simulink model "DFADAS2_SenFus_v1_201204RC_training_210115"  (R2018b)
settings: Solver=FixedStepDiscrete  StartTime=0.0  StopTime=inf  FixedStep=0.002  RelTol=1e-3  EnableMultiTasking=on
PreLoadFcn:
  | RTWConfigurationCB('preloadfcn', bdroot);
libraries: canmsglib x108, simulink x48, canfdmsglib x12
(part 9 of 28)

== system DFADAS2_SenFus_v1_201204RC_training_210115/Signal Input (Input)/Signal Input (50ms) (Input50)/Cmr/CmrInfo ==
  note: Level: 3
  Bus Creator : BusCreator  Inputs=6
  Bus Creator1 : BusCreator  Inputs=6
  Bus Creator2 : BusCreator  Inputs=5
  Bus Creator3 : BusCreator  Inputs=5
  Bus Creator4 : BusCreator  Inputs=4
  Bus Creator5 : BusCreator  Inputs=4
  "L0 Information (L0Info) " : Subsystem
  L1 Information (L1Info) : Subsystem
  R0 Information (R0Info) : Subsystem
  R1 Information (R1Info) : Subsystem
  LaneRx_bsLaneInfo : Outport
  LaneRx_efLanesFaultSyn : Outport  Port=2
  wires:
  Bus Creator/1 -> Bus Creator4/1  "CmrRxPrcs_bsL0Info"
  Bus Creator5/1 -> LaneRx_efLanesFaultSyn/1
  L1 Information (L1Info)/6(L1Info_efL1FaultSyn) -> Bus Creator5/3  "CmrRxPrcs_efL1FaultSyn"
  R0 Information (R0Info)/6(R0Info_facmR0Rng) -> Bus Creator1/6  "CmrRxPrcs_facmR0Rng"
  R1 Information (R1Info)/6(R0Info_efR0FaultSyn) -> Bus Creator5/4  "CmrRxPrcs_efR1FaultSyn"
  Bus Creator4/1 -> LaneRx_bsLaneInfo/1
  "L0 Information (L0Info) "/6(L0Info_facmL0Rng) -> Bus Creator/6  "CmrRxPrcs_facmL0Rng"
  R0 Information (R0Info)/4(R0Info_facmR0C3) -> Bus Creator1/4  "CmrRxPrcs_facmR0C3"
  R1 Information (R1Info)/1(R0Info_facmR0C0) -> Bus Creator3/1  "CmrRxPrcs_facmR1C0"
  R0 Information (R0Info)/3(R0Info_facmR0C2) -> Bus Creator1/3  "CmrRxPrcs_facmR0C2"
  "L0 Information (L0Info) "/4(L0Info_facmL0C3) -> Bus Creator/4  "CmrRxPrcs_facmL0C3"
  Bus Creator3/1 -> Bus Creator4/4  "CmrRxPrcs_bsR1Info"
  R0 Information (R0Info)/1(R0Info_facmR0C0) -> Bus Creator1/1  "CmrRxPrcs_facmR0C0"
  L1 Information (L1Info)/5(L1Info_facmL1Ql) -> Bus Creator2/5  "CmrRxPrcs_facmL1Ql"
  L1 Information (L1Info)/4(L1Info_facmL1C3) -> Bus Creator2/4  "CmrRxPrcs_facmL1C3"
  L1 Information (L1Info)/3(L1Info_facmL1C2) -> Bus Creator2/3  "CmrRxPrcs_facmL1C2"
  R0 Information (R0Info)/7(R0Info_efR0FaultSyn) -> Bus Creator5/2  "CmrRxPrcs_efR0FaultSyn"
  L1 Information (L1Info)/2(L1Info_facmL1C1) -> Bus Creator2/2  "CmrRxPrcs_facmL1C1"
  "L0 Information (L0Info) "/7(L0Info_efL0FaultSyn) -> Bus Creator5/1  "CmrRxPrcs_efL0FaultSyn"
  "L0 Information (L0Info) "/3(L0Info_facmL0C2) -> Bus Creator/3  "CmrRxPrcs_facmL0C2"
  R1 Information (R1Info)/4(R0Info_facmR0C3) -> Bus Creator3/4  "CmrRxPrcs_facmR1C3"
  R1 Information (R1Info)/2(R0Info_facmR0C1) -> Bus Creator3/2  "CmrRxPrcs_facmR1C1"
  Bus Creator2/1 -> Bus Creator4/3  "CmrRxPrcs_bsL1Info"
  R1 Information (R1Info)/3(R0Info_facmR0C2) -> Bus Creator3/3  "CmrRxPrcs_facmR1C2"
  "L0 Information (L0Info) "/1(L0Info_facmL0C0) -> Bus Creator/1  "CmrRxPrcs_facmL0C0"
  R0 Information (R0Info)/5(R0Info_facmR0Ql) -> Bus Creator1/5  "CmrRxPrcs_facmR0Ql"
  L1 Information (L1Info)/1(L1Info_facmL1C0) -> Bus Creator2/1  "CmrRxPrcs_facmL1C0"
  "L0 Information (L0Info) "/5(L0Info_facmL0Ql) -> Bus Creator/5  "CmrRxPrcs_facmL0Ql"
  "L0 Information (L0Info) "/2(L0Info_facmL0C1) -> Bus Creator/2  "CmrRxPrcs_facmL0C1"
  R1 Information (R1Info)/5(R0Info_facmR0Ql) -> Bus Creator3/5  "CmrRxPrcs_facmR1Ql"
  Bus Creator1/1 -> Bus Creator4/2  "CmrRxPrcs_bsR0Info"
  R0 Information (R0Info)/2(R0Info_facmR0C1) -> Bus Creator1/2  "CmrRxPrcs_facmR0C1"

== system DFADAS2_SenFus_v1_201204RC_training_210115/Signal Input (Input)/Signal Input (50ms) (Input50)/Front Left Radar(S2) Objects Information (FLRdr)/S0 Data Frame Read ==
  note: 目标：
      | ① 将可见的数据帧全部读出；
      | ② 仅对最新可见VF的数据帧进行数据解析。
      |
      | 首先将旧VF帧读完（不解析），然后进行RemainderCnt+1次的读取。最后一次读取的数据不解析，用于为未收到信号的通道置零。
  HFVFCnt : Inport
  IC : Inport  Port=2
  ObjectNum : Inport  Port=3
  Compare To Constant : simulink/Logic and Bit Operations/Compare To Constant  relop=>  const=0  OutDataTypeStr=boolean
  Enabled Subsystem : Subsystem  TreatAsAtomicUnit=on
  Logical Operator1 : Logic  Operator=OR  AllPortsSameDT=off  OutDataTypeStr=boolean
  Logical Operator3 : Logic  AllPortsSameDT=off  OutDataTypeStr=boolean
  Relational Operator3 : RelationalOperator  Operator===  OutDataTypeStr=boolean  RndMeth=Simplest
  S-Function200 : S-Function  FunctionName=NSTC297CANFDReceiveBlkLib  Parameters=|  SFunctionDeploymentMode=off  EnableBusSupport=off  mask(NSTC297 CANFD Receive){Ns_DeviceID=General Control Unit Gen2, Ns_ChannelNum=1, Ns_FrameID=855, Ns_IsVirtualFrame=on, Ns_RoleInVirtualFrame=Data Frame, Ns_HeaderFrameID=854, Ns_VirtualFrameStatusFlg=off, Ns_IncompleteFrameCntFlg=off, Ns_OverflowCntFlg=off, Ns_FrameBufferSize=5, Ns_SampleTime=-1}
      | uint16(Ns_DeviceID),
      | uint16(Ns_ChannelNum),
      | uint32(Ns_FrameID),
      | uint8(Ns_IsVirtualFrame),
      | uint16(Ns_RoleInVirtualFrame),
      | uint32(Ns_HeaderFrameID),
      | uint8(Ns_VirtualFrameStatusFlg),
      | uint8(Ns_IncompleteFrameCntFlg),
      | uint8(Ns_OverflowCntFlg),
      | uint16(Ns_FrameBufferSize),
      | double(Ns_SampleTime)
      mask prompts: Ns_DeviceID "Device:"; Ns_ChannelNum "Channel number:"; Ns_FrameID "Frame ID:"; Ns_IsVirtualFrame "Belong to a virtual frame"; Ns_RoleInVirtualFrame "Position in virtual frame:"; Ns_HeaderFrameID "Header frame ID:"; Ns_VirtualFrameStatusFlg "Current virtural frame status output"; Ns_IncompleteFrameCntFlg "Incomplete virtual frame count output"; Ns_OverflowCntFlg "Overflow count output"; Ns_FrameBufferSize "Frame buffer size:"; Ns_SampleTime "Sample time:"
      mask init:
      | NSTC297CANFDReceive_callback('portlabels');
      mask TypeOptions Ns_DeviceID: General Control Unit Gen2 | ADAS Control Unit Gen2
      mask TypeOptions Ns_ChannelNum: 0 | 1 | 2 | 3 | 4 | 5
      mask Callback Ns_IsVirtualFrame: NSTC297CANFDReceive_callback('Belong to a virtual frame');
      mask TypeOptions Ns_RoleInVirtualFrame: Header Frame | Data Frame | Trailer Frame
      mask Callback Ns_RoleInVirtualFrame: NSTC297CANFDReceive_callback('Position in virtual frame');
      mask Display: color('blue');text(0.02,0.9,'NovSteeds TC297','horizontalAlignment','left');color('blue');text(0.5,0.7,'CANFD Receive','horizontalAlignment','center');color('black');text(0.5,0.6,'Channel: 1','horizontalAlignment','center');text(0.5,0.5,'ID: 855','horizontalAlignment','center');text(0.5,0.4,'Virtual Frame: Data Frame','horizontalAlignment','center');port_label('output',1, 'VFCnt');port_label('output',2, 'RemainderCnt');port_label('output',3, 'Msg');
  Subsystem : Subsystem
  Switch : Switch  Criteria=u2 > Threshold
  VsblMnmt : Subsystem
  While Iterator : WhileIterator  MaxIters=10  ResetStates=reset
  RLRdr_bsObjInfo : Outport
  wires:
  Switch/1 -> RLRdr_bsObjInfo/1
  ObjectNum/1 -> Switch/2, Enabled Subsystem/3(obj_num)
  Logical Operator3/1 -> Enabled Subsystem/Enable, Logical Operator1/2
  Subsystem/1(RLRdrObjInfo) -> Switch/3
  Enabled Subsystem/1(RLRdrObjInfo) -> Switch/1
  Compare To Constant/1 -> Logical Operator3/2
  Relational Operator3/1 -> Logical Operator3/1
  Logical Operator1/1 -> While Iterator/1
  VsblMnmt/1(EnFlg) -> Logical Operator1/1
  HFVFCnt/1 -> Relational Operator3/1, VsblMnmt/1(HFVFCnt)
  S-Function200/1 -> Relational Operator3/2, VsblMnmt/2(LocVFCnt)
  S-Function200/2 -> Enabled Subsystem/1(RemainderCnt), Compare To Constant/1
  S-Function200/3 -> Enabled Subsystem/2(Msg)
  IC/1 -> While Iterator/2

== system DFADAS2_SenFus_v1_201204RC_training_210115/Signal Input (Input)/Signal Input (50ms) (Input50)/Front Left Radar(S2) Objects Information (FLRdr)/S0 Header Frame Read ==
  note: 目标：
      | ① 将缓冲中的全部数据读出；
      | ② 仅对最后一帧进行解析
  IC : Inport
  Compare To Constant : simulink/Logic and Bit Operations/Compare To Constant  relop=>  const=0  OutDataTypeStr=boolean
  Compare To Constant1 : simulink/Logic and Bit Operations/Compare To Constant  relop===  const=1  OutDataTypeStr=boolean
  Enabled Subsystem : Subsystem  TreatAsAtomicUnit=on
  S-Function100 : S-Function  FunctionName=NSTC297CANFDReceiveBlkLib  Parameters=|  SFunctionDeploymentMode=off  EnableBusSupport=off  mask(NSTC297 CANFD Receive){Ns_DeviceID=General Control Unit Gen2, Ns_ChannelNum=1, Ns_FrameID=854, Ns_IsVirtualFrame=on, Ns_RoleInVirtualFrame=Header Frame, Ns_HeaderFrameID=0, Ns_VirtualFrameStatusFlg=off, Ns_IncompleteFrameCntFlg=off, Ns_OverflowCntFlg=off, Ns_FrameBufferSize=5, Ns_SampleTime=-1}
      | uint16(Ns_DeviceID),
      | uint16(Ns_ChannelNum),
      | uint32(Ns_FrameID),
      | uint8(Ns_IsVirtualFrame),
      | uint16(Ns_RoleInVirtualFrame),
      | uint32(Ns_HeaderFrameID),
      | uint8(Ns_VirtualFrameStatusFlg),
      | uint8(Ns_IncompleteFrameCntFlg),
      | uint8(Ns_OverflowCntFlg),
      | uint16(Ns_FrameBufferSize),
      | double(Ns_SampleTime)
      mask prompts: Ns_DeviceID "Device:"; Ns_ChannelNum "Channel number:"; Ns_FrameID "Frame ID:"; Ns_IsVirtualFrame "Belong to a virtual frame"; Ns_RoleInVirtualFrame "Position in virtual frame:"; Ns_HeaderFrameID "Header frame ID:"; Ns_VirtualFrameStatusFlg "Current virtural frame status output"; Ns_IncompleteFrameCntFlg "Incomplete virtual frame count output"; Ns_OverflowCntFlg "Overflow count output"; Ns_FrameBufferSize "Frame buffer size:"; Ns_SampleTime "Sample time:"
      mask init:
      | NSTC297CANFDReceive_callback('portlabels');
      mask TypeOptions Ns_DeviceID: General Control Unit Gen2 | ADAS Control Unit Gen2
      mask TypeOptions Ns_ChannelNum: 0 | 1 | 2 | 3 | 4 | 5
      mask Callback Ns_IsVirtualFrame: NSTC297CANFDReceive_callback('Belong to a virtual frame');
      mask TypeOptions Ns_RoleInVirtualFrame: Header Frame | Data Frame | Trailer Frame
      mask Callback Ns_RoleInVirtualFrame: NSTC297CANFDReceive_callback('Position in virtual frame');
      mask Display: color('blue');text(0.02,0.9,'NovSteeds TC297','horizontalAlignment','left');color('blue');text(0.5,0.7,'CANFD Receive','horizontalAlignment','center');color('black');text(0.5,0.6,'Channel: 1','horizontalAlignment','center');text(0.5,0.5,'ID: 854','horizontalAlignment','center');text(0.5,0.4,'Virtual Frame: Header Frame','horizontalAlignment','center');port_label('output',1, 'VFCnt');port_label('output',2, 'RemainderCnt');port_label('output',3, 'Msg');
  While Iterator : WhileIterator  MaxIters=10  ResetStates=reset
  RLRdr_bsCmnInfo : Outport
  HFVFCnt : Outport  Port=2
  wires:
  S-Function100/1 -> HFVFCnt/1
  Compare To Constant1/1 -> Enabled Subsystem/Enable
  S-Function100/2 -> Compare To Constant1/1, Compare To Constant/1
  Enabled Subsystem/1(Sigs) -> RLRdr_bsCmnInfo/1
  S-Function100/3 -> Enabled Subsystem/1(Msg)
  Compare To Constant/1 -> While Iterator/1
  IC/1 -> While Iterator/2

== system DFADAS2_SenFus_v1_201204RC_training_210115/Signal Input (Input)/Signal Input (50ms) (Input50)/Front Left Radar(S2) Objects Information (FLRdr)/S0 Trailer Frame Read ==
  HFVFCnt : Inport
  "IC " : Inport  Port=2
  S-Function300 : S-Function  FunctionName=NSTC297CANFDReceiveBlkLib  Parameters=|  SFunctionDeploymentMode=off  EnableBusSupport=off  mask(NSTC297 CANFD Receive){Ns_DeviceID=General Control Unit Gen2, Ns_ChannelNum=1, Ns_FrameID=856, Ns_IsVirtualFrame=on, Ns_RoleInVirtualFrame=Trailer Frame, Ns_HeaderFrameID=854, Ns_VirtualFrameStatusFlg=off, Ns_IncompleteFrameCntFlg=off, Ns_OverflowCntFlg=off, Ns_FrameBufferSize=5, Ns_SampleTime=-1}
      | uint16(Ns_DeviceID),
      | uint16(Ns_ChannelNum),
      | uint32(Ns_FrameID),
      | uint8(Ns_IsVirtualFrame),
      | uint16(Ns_RoleInVirtualFrame),
      | uint32(Ns_HeaderFrameID),
      | uint8(Ns_VirtualFrameStatusFlg),
      | uint8(Ns_IncompleteFrameCntFlg),
      | uint8(Ns_OverflowCntFlg),
      | uint16(Ns_FrameBufferSize),
      | double(Ns_SampleTime)
      mask prompts: Ns_DeviceID "Device:"; Ns_ChannelNum "Channel number:"; Ns_FrameID "Frame ID:"; Ns_IsVirtualFrame "Belong to a virtual frame"; Ns_RoleInVirtualFrame "Position in virtual frame:"; Ns_HeaderFrameID "Header frame ID:"; Ns_VirtualFrameStatusFlg "Current virtural frame status output"; Ns_IncompleteFrameCntFlg "Incomplete virtual frame count output"; Ns_OverflowCntFlg "Overflow count output"; Ns_FrameBufferSize "Frame buffer size:"; Ns_SampleTime "Sample time:"
      mask init:
      | NSTC297CANFDReceive_callback('portlabels');
      mask TypeOptions Ns_DeviceID: General Control Unit Gen2 | ADAS Control Unit Gen2
      mask TypeOptions Ns_ChannelNum: 0 | 1 | 2 | 3 | 4 | 5
      mask Callback Ns_IsVirtualFrame: NSTC297CANFDReceive_callback('Belong to a virtual frame');
      mask TypeOptions Ns_RoleInVirtualFrame: Header Frame | Data Frame | Trailer Frame
      mask Callback Ns_RoleInVirtualFrame: NSTC297CANFDReceive_callback('Position in virtual frame');
      mask Display: color('blue');text(0.02,0.9,'NovSteeds TC297','horizontalAlignment','left');color('blue');text(0.5,0.7,'CANFD Receive','horizontalAlignment','center');color('black');text(0.5,0.6,'Channel: 1','horizontalAlignment','center');text(0.5,0.5,'ID: 856','horizontalAlignment','center');text(0.5,0.4,'Virtual Frame: Trailer Frame','horizontalAlignment','center');port_label('output',1, 'VFCnt');port_label('output',2, 'RemainderCnt');port_label('output',3, 'Msg');
  Terminator1 : Terminator
  Terminator2 : Terminator
  VsblMnmt : Subsystem
  While Iterator : WhileIterator  MaxIters=10  ResetStates=reset
  wires:
  VsblMnmt/1(EnFlg) -> While Iterator/1
  S-Function300/1 -> VsblMnmt/2(LocVFCnt)
  HFVFCnt/1 -> VsblMnmt/1(HFVFCnt)
  S-Function300/2 -> Terminator2/1
  S-Function300/3 -> Terminator1/1
  "IC "/1 -> While Iterator/2

== system DFADAS2_SenFus_v1_201204RC_training_210115/Signal Input (Input)/Signal Input (50ms) (Input50)/Front Left Radar(S2) Objects Information (FLRdr)/Subsystem ==
  In1 : Inport
  Bus Selector : BusSelector  OutputSignals=FLRdr_bsObjInfo.M00ObjInfo,FLRdr_bsObjInfo.M01ObjInfo,FLRdr_bsObjInfo.M10ObjInfo,FLRdr_bsObjInfo.M11ObjInfo,FLRdr_bsObjInfo.M20ObjInfo,FLRdr_bsObjInfo.M21ObjInfo,FLRdr_bsObjInfo.M30ObjInfo,FLRdr_bsObjInfo.M31ObjInfo,FLRdr_bsObjInfo.M40ObjInfo,FLRdr_bsObjInfo.M41ObjInfo,FLRdr_bsCmnInfo
  Bus Selector1 : BusSelector  OutputSignals=Id_S0_001,XPos_S0_001,YPos_S0_001
  Bus Selector10 : BusSelector  OutputSignals=Id_S0_008,XPos_S0_008,YPos_S0_008
  Bus Selector11 : BusSelector  OutputSignals=Id_S0_009,XPos_S0_009,YPos_S0_009
  Bus Selector2 : BusSelector  OutputSignals=Id_S0_002,XPos_S0_002,YPos_S0_002
  Bus Selector3 : BusSelector  OutputSignals=Id_S0_003,XPos_S0_003,YPos_S0_003
  Bus Selector4 : BusSelector  OutputSignals=Id_S0_004,XPos_S0_004,YPos_S0_004
  Bus Selector5 : BusSelector  OutputSignals=Id_S0_005,XPos_S0_005,YPos_S0_005
  Bus Selector6 : BusSelector  OutputSignals=NumberOfObjects_S2
  Bus Selector7 : BusSelector  OutputSignals=Id_S0_010,XPos_S0_010,YPos_S0_010
  Bus Selector8 : BusSelector  OutputSignals=Id_S0_006,XPos_S0_006,YPos_S0_006
  Bus Selector9 : BusSelector  OutputSignals=Id_S0_007,XPos_S0_007,YPos_S0_007
  CAN FD Pack : canfdmsglib/CAN FD Pack  MsgList=(none)  MsgName=Msg  ProtocolMode=CAN FD  MsgIDType=Standard (11-bit identifier)  MsgIdentifier=1634  MsgLength=64  SignalInfo=Signal1$0$16$1$2$1$0$1$0$0$Inf$#Signal2$16$16$1$2$1$0$0.05$-400$-Inf$Inf$#Signal3$32$16$1$2$1$0$0.01$-80$-Inf$Inf$#Signal4$48$16$1$2$1$0$1$0$0$Inf$#Signal5$64$16$1$2$1$0$0.05$-400$-Inf$Inf$#Signal6$80$16$1$2$1$0$0.01$-80$-Inf$Inf$#Signal7$96$16$1$2$1$0$1$0$0$Inf$#Signal8$112$16$1$2$1$0$0.05$-400$-Inf$Inf$#Signal9$128$16$1$2$1$0$0.01$-80$-Inf$Inf$#Signal10$144$16$1$2$1$0$1$0$0$Inf$#Signal11$160$16$1$2$1$0$0.05$-400$-Inf$Inf$#Signal12$176$16$1$2$1$0$0.01$-80$-Inf$Inf$#Signal13$192$16$1$2$1$0$1$0$0$Inf$#Signal14$208$16$1$2$1$0$0.05$-400$-Inf$Inf$#Signal15$224$16$1$2$1$0$0.01$-80$-Inf$Inf$#Signal16$240$16$1$2$1$0$1$0$0$Inf$#Signal17$256$16$1$2$1$0$0.05$-400$-Inf$Inf$#Signal18$272$16$1$2$1$0$0.01$-80$-Inf$Inf$#Signal19$288$16$1$2$1$0$1$0$0$Inf$#Signal20$304$16$1$2$1$0$0.05$-400$-Inf$Inf$#Signal21$320$16$1$2$1$0$0.01$-80$-Inf$Inf$#Signal22$336$16$1$2$1$0$1$0$0$Inf$#Signal23$352$16$1$2$1$0$0.05$-400$-Inf$Inf$#Signal24$368$16$1$2$1$0$0.01$-80$-Inf$Inf$#Signal25$384$16$1$2$1$0$1$0$0$Inf$#Signal26$400$16$1$2$1$0$0.05$-400$-Inf$Inf$#Signal27$416$16$1$2$1$0$0.01$-80$-Inf$Inf$#Signal28$432$16$1$2$1$0$1$0$0$Inf$#Signal29$448$16$1$2$1$0$0.05$-400$-Inf$Inf$#Signal30$464$16$1$2$1$0$0.01$-80$-Inf$Inf$#num_obj$480$16$1$2$1$0$1$0$0$Inf$#m_value$496$16$1$2$1$0$1$0$0$Inf$#  NSignals=32  StartBits=str2num('[int32(0);int32(16);int32(32);int32(48);int32(64);int32(80);int32(96);int32(112);int32(128);int32(144);int32(160);int32(176);int32(192);int32(208);int32(224);int32(240);int32(256);int32(272);int32(288);int32(304);int32(320);int32(336);int32(352);int32(368);int32(384);int32(400);int32(416);int32(432);int32(448);int32(464);int32(480);int32(496)]')  SignalSizes=str2num('[int32(16);int32(16);int32(16);int32(16);int32(16);int32(16);int32(16);int32(16);int32(16);int32(16);int32(16);int32(16);int32(16);int32(16);int32(16);int32(16);int32(16);int32(16);int32(16);int32(16);int32(16);int32(16);int32(16);int32(16);int32(16);int32(16);int32(16);int32(16);int32(16);int32(16);int32(16);int32(16)]')  ByteOrders=str2num('[int32(1);int32(1);int32(1);int32(1);int32(1);int32(1);int32(1);int32(1);int32(1);int32(1);int32(1);int32(1);int32(1);int32(1);int32(1);int32(1);int32(1);int32(1);int32(1);int32(1);int32(1);int32(1);int32(1);int32(1);int32(1);int32(1);int32(1);int32(1);int32(1);int32(1);int32(1);int32(1)]')  DataTypes=str2num('[int32(2);int32(2);int32(2);int32(2);int32(2);int32(2);int32(2);int32(2);int32(2);int32(2);int32(2);int32(2);int32(2);int32(2);int32(2);int32(2);int32(2);int32(2);int32(2);int32(2);int32(2);int32(2);int32(2);int32(2);int32(2);int32(2);int32(2);int32(2);int32(2);int32(2);int32(2);int32(2)]')  MultiplexTypes=str2num('[int32(1);int32(1);int32(1);int32(1);int32(1);int32(1);int32(1);int32(1);int32(1);int32(1);int32(1);int32(1);int32(1);int32(1);int32(1);int32(1);int32(1);int32(1);int32(1);int32(1);int32(1);int32(1);int32(1);int32(1);int32(1);int32(1);int32(1);int32(1);int32(1);int32(1);int32(1);int32(1)]')  MultiplexValues=str2num('[double(0);double(0);double(0);double(0);double(0);double(0);double(0);double(0);double(0);double(0);double(0);double(0);double(0);double(0);double(0);double(0);double(0);double(0);double(0);double(0);double(0);double(0);double(0);double(0);double(0);double(0);double(0);double(0);double(0);double(0);double(0);double(0)]')  Factors=str2num('[double(1);double(0.05);double(0.01);double(1);double(0.05);double(0.01);double(1);double(0.05);double(0.01);double(1);double(0.05);double(0.01);double(1);double(0.05);double(0.01);double(1);double(0.05);double(0.01);double(1);double(0.05);double(0.01);double(1);double(0.05);double(0.01);double(1);double(0.05);double(0.01);double(1);double(0.05);double(0.01);double(1);double(1)]')  Offsets=str2num('[double(0);double(-400);double(-80);double(0);double(-400);double(-80);double(0);double(-400);double(-80);double(0);double(-400);double(-80);double(0);double(-400);double(-80);double(0);double(-400);double(-80);double(0);double(-400);double(-80);double(0);double(-400);double(-80);double(0);double(-400);double(-80);double(0);double(-400);double(-80);double(0);double(0)]')  Minimums=str2num('[double(0);double(-Inf);double(-Inf);double(0);double(-Inf);double(-Inf);double(0);double(-Inf);double(-Inf);double(0);double(-Inf);double(-Inf);double(0);double(-Inf);double(-Inf);double(0);double(-Inf);double(-Inf);double(0);double(-Inf);double(-Inf);double(0);double(-Inf);double(-Inf);double(0);double(-Inf);double(-Inf);double(0);double(-Inf);double(-Inf);double(0);double(0)]')  Maximums=str2num('[double(Inf);double(Inf);double(Inf);double(Inf);double(Inf);double(Inf);double(Inf);double(Inf);double(Inf);double(Inf);double(Inf);double(Inf);double(Inf);double(Inf);double(Inf);double(Inf);double(Inf);double(Inf);double(Inf);double(Inf);double(Inf);double(Inf);double(Inf);double(Inf);double(Inf);double(Inf);double(Inf);double(Inf);double(Inf);double(Inf);double(Inf);double(Inf)]')  Remote=off  ApplyMinMax=off  BRSSwitch=off
      settings: SourceProductName=Simulink Real-Time  DataFormat=manually specified signals
  S-Function9 : S-Function  FunctionName=NSTC297CANFDTransmitBlkLib  Parameters=|  SFunctionDeploymentMode=off  EnableBusSupport=off  mask(NSTC297 CANFD Transmit){Ns_DeviceID=ADAS Control Unit Gen2, Ns_ChannelNum=3, Ns_FrameType=CANFD, Ns_FrameBufferSize=0, Ns_OverflowCntOutFlg=off, Ns_SampleTime=-1}
      | uint16(Ns_DeviceID),
      | uint16(Ns_ChannelNum),
      | uint16(Ns_FrameType),
      | uint16(Ns_FrameBufferSize),
      | uint8(Ns_OverflowCntOutFlg),
      | double(Ns_SampleTime)
      mask prompts: Ns_DeviceID "Device:"; Ns_ChannelNum "Channel number:"; Ns_FrameType "Frame type:"; Ns_FrameBufferSize "Frame buffer size:"; Ns_OverflowCntOutFlg "Overflow count output"; Ns_SampleTime "Sample time:"
      mask init:
      | NSTC297CANFDTransmit_callback('portlabels');
      mask TypeOptions Ns_DeviceID: General Control Unit Gen2 | ADAS Control Unit Gen2
      mask TypeOptions Ns_ChannelNum: 0 | 1 | 2 | 3 | 4 | 5
      mask TypeOptions Ns_FrameType: CAN | CANFD
      mask Display: color('blue');text(0.98,0.9,'NovSteeds TC297','horizontalAlignment','right');color('blue');text(0.5,0.65,'CANFD Transmit','horizontalAlignment','center');color('black');text(0.5,0.35,'Type: CANFD','horizontalAlignment','center');text(0.5,0.50,'Channel: 3','horizontalAlignment','center');port_label('input',1, 'Msg');
  wires:
  Bus Selector/2 -> Bus Selector2/1  "<M01ObjInfo>"
  Bus Selector7/1 -> CAN FD Pack/28  "<Id_S0_010>"
  Bus Selector/11 -> Bus Selector6/1  "<FLRdr_bsCmnInfo>"
  Bus Selector6/1 -> CAN FD Pack/31  "<NumberOfObjects_S2>"
  Bus Selector8/3 -> CAN FD Pack/18  "<YPos_S0_006>"
  Bus Selector3/2 -> CAN FD Pack/8  "<XPos_S0_003>"
  Bus Selector7/3 -> CAN FD Pack/30  "<YPos_S0_010>"
  Bus Selector3/3 -> CAN FD Pack/9  "<YPos_S0_003>"
  Bus Selector9/3 -> CAN FD Pack/21  "<YPos_S0_007>"
  Bus Selector2/1 -> CAN FD Pack/4  "<Id_S0_002>"
  Bus Selector7/2 -> CAN FD Pack/29  "<XPos_S0_010>"
  Bus Selector10/1 -> CAN FD Pack/22  "<Id_S0_008>"
  In1/1 -> Bus Selector/1
  Bus Selector11/2 -> CAN FD Pack/26  "<XPos_S0_009>"
  Bus Selector10/2 -> CAN FD Pack/23  "<XPos_S0_008>"
  Bus Selector4/3 -> CAN FD Pack/12  "<YPos_S0_004>"
  Bus Selector2/3 -> CAN FD Pack/6  "<YPos_S0_002>"
  Bus Selector4/2 -> CAN FD Pack/11  "<XPos_S0_004>"
  Bus Selector1/1 -> CAN FD Pack/1  "<Id_S0_001>"
  CAN FD Pack/1 -> S-Function9/1
  Bus Selector8/1 -> CAN FD Pack/16  "<Id_S0_006>"
  Bus Selector5/2 -> CAN FD Pack/14  "<XPos_S0_005>"
  Bus Selector2/2 -> CAN FD Pack/5  "<XPos_S0_002>"
  Bus Selector11/3 -> CAN FD Pack/27  "<YPos_S0_009>"
  Bus Selector3/1 -> CAN FD Pack/7  "<Id_S0_003>"
  Bus Selector/6 -> Bus Selector8/1  "<M21ObjInfo>"
  Bus Selector5/3 -> CAN FD Pack/15  "<YPos_S0_005>"
  Bus Selector4/1 -> CAN FD Pack/10  "<Id_S0_004>"
  Bus Selector10/3 -> CAN FD Pack/24  "<YPos_S0_008>"
  Bus Selector/7 -> Bus Selector9/1  "<M30ObjInfo>"
  Bus Selector1/3 -> CAN FD Pack/3  "<YPos_S0_001>"
  Bus Selector/1 -> Bus Selector1/1  "<M00ObjInfo>"
  Bus Selector/9 -> Bus Selector11/1  "<M40ObjInfo>"
  Bus Selector/8 -> Bus Selector10/1  "<M31ObjInfo>"
  Bus Selector9/1 -> CAN FD Pack/19  "<Id_S0_007>"
  Bus Selector9/2 -> CAN FD Pack/20  "<XPos_S0_007>"
  Bus Selector/3 -> Bus Selector3/1  "<M10ObjInfo>"
  Bus Selector/5 -> Bus Selector5/1  "<M20ObjInfo>"
  Bus Selector/4 -> Bus Selector4/1  "<M11ObjInfo>"
  Bus Selector1/2 -> CAN FD Pack/2  "<XPos_S0_001>"
  Bus Selector5/1 -> CAN FD Pack/13  "<Id_S0_005>"
  Bus Selector11/1 -> CAN FD Pack/25  "<Id_S0_009>"
  Bus Selector8/2 -> CAN FD Pack/17  "<XPos_S0_006>"
  Bus Selector/10 -> Bus Selector7/1  "<M41ObjInfo>"

== system DFADAS2_SenFus_v1_201204RC_training_210115/Signal Input (Input)/Signal Input (50ms) (Input50)/Front Right Radar(S3) Objects Information (FRRdr)/S0 Data Frame Read ==
  note: 目标：
      | ① 将可见的数据帧全部读出；
      | ② 仅对最新可见VF的数据帧进行数据解析。
      |
      | 首先将旧VF帧读完（不解析），然后进行RemainderCnt+1次的读取。最后一次读取的数据不解析，用于为未收到信号的通道置零。
  HFVFCnt : Inport
  IC : Inport  Port=2
  ObjectNum : Inport  Port=3
  Compare To Constant : simulink/Logic and Bit Operations/Compare To Constant  relop=>  const=0  OutDataTypeStr=boolean
  Enabled Subsystem : Subsystem  TreatAsAtomicUnit=on
  Logical Operator1 : Logic  Operator=OR  AllPortsSameDT=off  OutDataTypeStr=boolean
  Logical Operator3 : Logic  AllPortsSameDT=off  OutDataTypeStr=boolean
  Relational Operator3 : RelationalOperator  Operator===  OutDataTypeStr=boolean  RndMeth=Simplest
  S-Function200 : S-Function  FunctionName=NSTC297CANFDReceiveBlkLib  Parameters=|  SFunctionDeploymentMode=off  EnableBusSupport=off  mask(NSTC297 CANFD Receive){Ns_DeviceID=General Control Unit Gen2, Ns_ChannelNum=1, Ns_FrameID=858, Ns_IsVirtualFrame=on, Ns_RoleInVirtualFrame=Data Frame, Ns_HeaderFrameID=857, Ns_VirtualFrameStatusFlg=off, Ns_IncompleteFrameCntFlg=off, Ns_OverflowCntFlg=off, Ns_FrameBufferSize=5, Ns_SampleTime=-1}
      | uint16(Ns_DeviceID),
      | uint16(Ns_ChannelNum),
      | uint32(Ns_FrameID),
      | uint8(Ns_IsVirtualFrame),
      | uint16(Ns_RoleInVirtualFrame),
      | uint32(Ns_HeaderFrameID),
      | uint8(Ns_VirtualFrameStatusFlg),
      | uint8(Ns_IncompleteFrameCntFlg),
      | uint8(Ns_OverflowCntFlg),
      | uint16(Ns_FrameBufferSize),
      | double(Ns_SampleTime)
      mask prompts: Ns_DeviceID "Device:"; Ns_ChannelNum "Channel number:"; Ns_FrameID "Frame ID:"; Ns_IsVirtualFrame "Belong to a virtual frame"; Ns_RoleInVirtualFrame "Position in virtual frame:"; Ns_HeaderFrameID "Header frame ID:"; Ns_VirtualFrameStatusFlg "Current virtural frame status output"; Ns_IncompleteFrameCntFlg "Incomplete virtual frame count output"; Ns_OverflowCntFlg "Overflow count output"; Ns_FrameBufferSize "Frame buffer size:"; Ns_SampleTime "Sample time:"
      mask init:
      | NSTC297CANFDReceive_callback('portlabels');
      mask TypeOptions Ns_DeviceID: General Control Unit Gen2 | ADAS Control Unit Gen2
      mask TypeOptions Ns_ChannelNum: 0 | 1 | 2 | 3 | 4 | 5
      mask Callback Ns_IsVirtualFrame: NSTC297CANFDReceive_callback('Belong to a virtual frame');
      mask TypeOptions Ns_RoleInVirtualFrame: Header Frame | Data Frame | Trailer Frame
      mask Callback Ns_RoleInVirtualFrame: NSTC297CANFDReceive_callback('Position in virtual frame');
      mask Display: color('blue');text(0.02,0.9,'NovSteeds TC297','horizontalAlignment','left');color('blue');text(0.5,0.7,'CANFD Receive','horizontalAlignment','center');color('black');text(0.5,0.6,'Channel: 1','horizontalAlignment','center');text(0.5,0.5,'ID: 858','horizontalAlignment','center');text(0.5,0.4,'Virtual Frame: Data Frame','horizontalAlignment','center');port_label('output',1, 'VFCnt');port_label('output',2, 'RemainderCnt');port_label('output',3, 'Msg');
  Subsystem : Subsystem
  Switch : Switch  Criteria=u2 > Threshold
  VsblMnmt : Subsystem
  While Iterator : WhileIterator  MaxIters=10  ResetStates=reset
  RLRdr_bsObjInfo : Outport
  wires:
  IC/1 -> While Iterator/2
  S-Function200/3 -> Enabled Subsystem/2(Msg)
  S-Function200/2 -> Compare To Constant/1, Enabled Subsystem/1(RemainderCnt)
  S-Function200/1 -> VsblMnmt/2(LocVFCnt), Relational Operator3/2
  HFVFCnt/1 -> VsblMnmt/1(HFVFCnt), Relational Operator3/1
  VsblMnmt/1(EnFlg) -> Logical Operator1/1
  Logical Operator1/1 -> While Iterator/1
  Relational Operator3/1 -> Logical Operator3/1
  Compare To Constant/1 -> Logical Operator3/2
  Enabled Subsystem/1(RLRdrObjInfo) -> Switch/1
  Subsystem/1(RLRdrObjInfo) -> Switch/3
  Logical Operator3/1 -> Logical Operator1/2, Enabled Subsystem/Enable
  ObjectNum/1 -> Enabled Subsystem/3(obj_num), Switch/2
  Switch/1 -> RLRdr_bsObjInfo/1

== system DFADAS2_SenFus_v1_201204RC_training_210115/Signal Input (Input)/Signal Input (50ms) (Input50)/Front Right Radar(S3) Objects Information (FRRdr)/S0 Header Frame Read ==
  note: 目标：
      | ① 将缓冲中的全部数据读出；
      | ② 仅对最后一帧进行解析
  IC : Inport
  Compare To Constant : simulink/Logic and Bit Operations/Compare To Constant  relop=>  const=0  OutDataTypeStr=boolean
  Compare To Constant1 : simulink/Logic and Bit Operations/Compare To Constant  relop===  const=1  OutDataTypeStr=boolean
  Enabled Subsystem : Subsystem  TreatAsAtomicUnit=on
  S-Function100 : S-Function  FunctionName=NSTC297CANFDReceiveBlkLib  Parameters=|  SFunctionDeploymentMode=off  EnableBusSupport=off  mask(NSTC297 CANFD Receive){Ns_DeviceID=General Control Unit Gen2, Ns_ChannelNum=1, Ns_FrameID=857, Ns_IsVirtualFrame=on, Ns_RoleInVirtualFrame=Header Frame, Ns_HeaderFrameID=0, Ns_VirtualFrameStatusFlg=off, Ns_IncompleteFrameCntFlg=off, Ns_OverflowCntFlg=off, Ns_FrameBufferSize=5, Ns_SampleTime=-1}
      | uint16(Ns_DeviceID),
      | uint16(Ns_ChannelNum),
      | uint32(Ns_FrameID),
      | uint8(Ns_IsVirtualFrame),
      | uint16(Ns_RoleInVirtualFrame),
      | uint32(Ns_HeaderFrameID),
      | uint8(Ns_VirtualFrameStatusFlg),
      | uint8(Ns_IncompleteFrameCntFlg),
      | uint8(Ns_OverflowCntFlg),
      | uint16(Ns_FrameBufferSize),
      | double(Ns_SampleTime)
      mask prompts: Ns_DeviceID "Device:"; Ns_ChannelNum "Channel number:"; Ns_FrameID "Frame ID:"; Ns_IsVirtualFrame "Belong to a virtual frame"; Ns_RoleInVirtualFrame "Position in virtual frame:"; Ns_HeaderFrameID "Header frame ID:"; Ns_VirtualFrameStatusFlg "Current virtural frame status output"; Ns_IncompleteFrameCntFlg "Incomplete virtual frame count output"; Ns_OverflowCntFlg "Overflow count output"; Ns_FrameBufferSize "Frame buffer size:"; Ns_SampleTime "Sample time:"
      mask init:
      | NSTC297CANFDReceive_callback('portlabels');
      mask TypeOptions Ns_DeviceID: General Control Unit Gen2 | ADAS Control Unit Gen2
      mask TypeOptions Ns_ChannelNum: 0 | 1 | 2 | 3 | 4 | 5
      mask Callback Ns_IsVirtualFrame: NSTC297CANFDReceive_callback('Belong to a virtual frame');
      mask TypeOptions Ns_RoleInVirtualFrame: Header Frame | Data Frame | Trailer Frame
      mask Callback Ns_RoleInVirtualFrame: NSTC297CANFDReceive_callback('Position in virtual frame');
      mask Display: color('blue');text(0.02,0.9,'NovSteeds TC297','horizontalAlignment','left');color('blue');text(0.5,0.7,'CANFD Receive','horizontalAlignment','center');color('black');text(0.5,0.6,'Channel: 1','horizontalAlignment','center');text(0.5,0.5,'ID: 857','horizontalAlignment','center');text(0.5,0.4,'Virtual Frame: Header Frame','horizontalAlignment','center');port_label('output',1, 'VFCnt');port_label('output',2, 'RemainderCnt');port_label('output',3, 'Msg');
  While Iterator : WhileIterator  MaxIters=10  ResetStates=reset
  RLRdr_bsCmnInfo : Outport
  HFVFCnt : Outport  Port=2
  wires:
  IC/1 -> While Iterator/2
  Compare To Constant/1 -> While Iterator/1
  S-Function100/3 -> Enabled Subsystem/1(Msg)
  Enabled Subsystem/1(Sigs) -> RLRdr_bsCmnInfo/1
  S-Function100/2 -> Compare To Constant/1, Compare To Constant1/1
  Compare To Constant1/1 -> Enabled Subsystem/Enable
  S-Function100/1 -> HFVFCnt/1

== system DFADAS2_SenFus_v1_201204RC_training_210115/Signal Input (Input)/Signal Input (50ms) (Input50)/Front Right Radar(S3) Objects Information (FRRdr)/S0 Trailer Frame Read ==
  HFVFCnt : Inport
  "IC " : Inport  Port=2
  S-Function300 : S-Function  FunctionName=NSTC297CANFDReceiveBlkLib  Parameters=|  SFunctionDeploymentMode=off  EnableBusSupport=off  mask(NSTC297 CANFD Receive){Ns_DeviceID=General Control Unit Gen2, Ns_ChannelNum=1, Ns_FrameID=859, Ns_IsVirtualFrame=on, Ns_RoleInVirtualFrame=Trailer Frame, Ns_HeaderFrameID=857, Ns_VirtualFrameStatusFlg=off, Ns_IncompleteFrameCntFlg=off, Ns_OverflowCntFlg=off, Ns_FrameBufferSize=5, Ns_SampleTime=-1}
      | uint16(Ns_DeviceID),
      | uint16(Ns_ChannelNum),
      | uint32(Ns_FrameID),
      | uint8(Ns_IsVirtualFrame),
      | uint16(Ns_RoleInVirtualFrame),
      | uint32(Ns_HeaderFrameID),
      | uint8(Ns_VirtualFrameStatusFlg),
      | uint8(Ns_IncompleteFrameCntFlg),
      | uint8(Ns_OverflowCntFlg),
      | uint16(Ns_FrameBufferSize),
      | double(Ns_SampleTime)
      mask prompts: Ns_DeviceID "Device:"; Ns_ChannelNum "Channel number:"; Ns_FrameID "Frame ID:"; Ns_IsVirtualFrame "Belong to a virtual frame"; Ns_RoleInVirtualFrame "Position in virtual frame:"; Ns_HeaderFrameID "Header frame ID:"; Ns_VirtualFrameStatusFlg "Current virtural frame status output"; Ns_IncompleteFrameCntFlg "Incomplete virtual frame count output"; Ns_OverflowCntFlg "Overflow count output"; Ns_FrameBufferSize "Frame buffer size:"; Ns_SampleTime "Sample time:"
      mask init:
      | NSTC297CANFDReceive_callback('portlabels');
      mask TypeOptions Ns_DeviceID: General Control Unit Gen2 | ADAS Control Unit Gen2
      mask TypeOptions Ns_ChannelNum: 0 | 1 | 2 | 3 | 4 | 5
      mask Callback Ns_IsVirtualFrame: NSTC297CANFDReceive_callback('Belong to a virtual frame');
      mask TypeOptions Ns_RoleInVirtualFrame: Header Frame | Data Frame | Trailer Frame
      mask Callback Ns_RoleInVirtualFrame: NSTC297CANFDReceive_callback('Position in virtual frame');
      mask Display: color('blue');text(0.02,0.9,'NovSteeds TC297','horizontalAlignment','left');color('blue');text(0.5,0.7,'CANFD Receive','horizontalAlignment','center');color('black');text(0.5,0.6,'Channel: 1','horizontalAlignment','center');text(0.5,0.5,'ID: 859','horizontalAlignment','center');text(0.5,0.4,'Virtual Frame: Trailer Frame','horizontalAlignment','center');port_label('output',1, 'VFCnt');port_label('output',2, 'RemainderCnt');port_label('output',3, 'Msg');
  Terminator1 : Terminator
  Terminator2 : Terminator
  VsblMnmt : Subsystem
  While Iterator : WhileIterator  MaxIters=10  ResetStates=reset
  wires:
  "IC "/1 -> While Iterator/2
  S-Function300/3 -> Terminator1/1
  S-Function300/2 -> Terminator2/1
  HFVFCnt/1 -> VsblMnmt/1(HFVFCnt)
  S-Function300/1 -> VsblMnmt/2(LocVFCnt)
  VsblMnmt/1(EnFlg) -> While Iterator/1

== system DFADAS2_SenFus_v1_201204RC_training_210115/Signal Input (Input)/Signal Input (50ms) (Input50)/Front Right Radar(S3) Objects Information (FRRdr)/Subsystem ==
  In1 : Inport
  Bus Selector12 : BusSelector  OutputSignals=FRRdr_bsObjInfo.M00ObjInfo,FRRdr_bsObjInfo.M01ObjInfo,FRRdr_bsObjInfo.M10ObjInfo,FRRdr_bsObjInfo.M11ObjInfo,FRRdr_bsObjInfo.M20ObjInfo,FRRdr_bsObjInfo.M21ObjInfo,FRRdr_bsObjInfo.M30ObjInfo,FRRdr_bsObjInfo.M31ObjInfo,FRRdr_bsObjInfo.M40ObjInfo,FRRdr_bsObjInfo.M41ObjInfo,FRRdr_bsCmnInfo
  Bus Selector13 : BusSelector  OutputSignals=Id_S0_001,XPos_S0_001,YPos_S0_001
  Bus Selector14 : BusSelector  OutputSignals=Id_S0_008,XPos_S0_008,YPos_S0_008
  Bus Selector15 : BusSelector  OutputSignals=Id_S0_009,XPos_S0_009,YPos_S0_009
  Bus Selector16 : BusSelector  OutputSignals=Id_S0_002,XPos_S0_002,YPos_S0_002
  Bus Selector17 : BusSelector  OutputSignals=Id_S0_003,XPos_S0_003,YPos_S0_003
  Bus Selector18 : BusSelector  OutputSignals=Id_S0_004,XPos_S0_004,YPos_S0_004
  Bus Selector19 : BusSelector  OutputSignals=Id_S0_005,XPos_S0_005,YPos_S0_005
  Bus Selector20 : BusSelector  OutputSignals=NumberOfObjects_S3
  Bus Selector21 : BusSelector  OutputSignals=Id_S0_010,XPos_S0_010,YPos_S0_010
  Bus Selector22 : BusSelector  OutputSignals=Id_S0_006,XPos_S0_006,YPos_S0_006
  Bus Selector23 : BusSelector  OutputSignals=Id_S0_007,XPos_S0_007,YPos_S0_007
  CAN FD Pack1 : canfdmsglib/CAN FD Pack  MsgList=(none)  MsgName=Msg  ProtocolMode=CAN FD  MsgIDType=Standard (11-bit identifier)  MsgIdentifier=1635  MsgLength=64  SignalInfo=Signal1$0$16$1$2$1$0$1$0$0$Inf$#Signal2$16$16$1$2$1$0$0.05$-400$-Inf$Inf$#Signal3$32$16$1$2$1$0$0.01$-80$-Inf$Inf$#Signal4$48$16$1$2$1$0$1$0$0$Inf$#Signal5$64$16$1$2$1$0$0.05$-400$-Inf$Inf$#Signal6$80$16$1$2$1$0$0.01$-80$-Inf$Inf$#Signal7$96$16$1$2$1$0$1$0$0$Inf$#Signal8$112$16$1$2$1$0$0.05$-400$-Inf$Inf$#Signal9$128$16$1$2$1$0$0.01$-80$-Inf$Inf$#Signal10$144$16$1$2$1$0$1$0$0$Inf$#Signal11$160$16$1$2$1$0$0.05$-400$-Inf$Inf$#Signal12$176$16$1$2$1$0$0.01$-80$-Inf$Inf$#Signal13$192$16$1$2$1$0$1$0$0$Inf$#Signal14$208$16$1$2$1$0$0.05$-400$-Inf$Inf$#Signal15$224$16$1$2$1$0$0.01$-80$-Inf$Inf$#Signal16$240$16$1$2$1$0$1$0$0$Inf$#Signal17$256$16$1$2$1$0$0.05$-400$-Inf$Inf$#Signal18$272$16$1$2$1$0$0.01$-80$-Inf$Inf$#Signal19$288$16$1$2$1$0$1$0$0$Inf$#Signal20$304$16$1$2$1$0$0.05$-400$-Inf$Inf$#Signal21$320$16$1$2$1$0$0.01$-80$-Inf$Inf$#Signal22$336$16$1$2$1$0$1$0$0$Inf$#Signal23$352$16$1$2$1$0$0.05$-400$-Inf$Inf$#Signal24$368$16$1$2$1$0$0.01$-80$-Inf$Inf$#Signal25$384$16$1$2$1$0$1$0$0$Inf$#Signal26$400$16$1$2$1$0$0.05$-400$-Inf$Inf$#Signal27$416$16$1$2$1$0$0.01$-80$-Inf$Inf$#Signal28$432$16$1$2$1$0$1$0$0$Inf$#Signal29$448$16$1$2$1$0$0.05$-400$-Inf$Inf$#Signal30$464$16$1$2$1$0$0.01$-80$-Inf$Inf$#num_obj$480$16$1$2$1$0$1$0$0$Inf$#m_value$496$16$1$2$1$0$1$0$0$Inf$#  NSignals=32  StartBits=str2num('[int32(0);int32(16);int32(32);int32(48);int32(64);int32(80);int32(96);int32(112);int32(128);int32(144);int32(160);int32(176);int32(192);int32(208);int32(224);int32(240);int32(256);int32(272);int32(288);int32(304);int32(320);int32(336);int32(352);int32(368);int32(384);int32(400);int32(416);int32(432);int32(448);int32(464);int32(480);int32(496)]')  SignalSizes=str2num('[int32(16);int32(16);int32(16);int32(16);int32(16);int32(16);int32(16);int32(16);int32(16);int32(16);int32(16);int32(16);int32(16);int32(16);int32(16);int32(16);int32(16);int32(16);int32(16);int32(16);int32(16);int32(16);int32(16);int32(16);int32(16);int32(16);int32(16);int32(16);int32(16);int32(16);int32(16);int32(16)]')  ByteOrders=str2num('[int32(1);int32(1);int32(1);int32(1);int32(1);int32(1);int32(1);int32(1);int32(1);int32(1);int32(1);int32(1);int32(1);int32(1);int32(1);int32(1);int32(1);int32(1);int32(1);int32(1);int32(1);int32(1);int32(1);int32(1);int32(1);int32(1);int32(1);int32(1);int32(1);int32(1);int32(1);int32(1)]')  DataTypes=str2num('[int32(2);int32(2);int32(2);int32(2);int32(2);int32(2);int32(2);int32(2);int32(2);int32(2);int32(2);int32(2);int32(2);int32(2);int32(2);int32(2);int32(2);int32(2);int32(2);int32(2);int32(2);int32(2);int32(2);int32(2);int32(2);int32(2);int32(2);int32(2);int32(2);int32(2);int32(2);int32(2)]')  MultiplexTypes=str2num('[int32(1);int32(1);int32(1);int32(1);int32(1);int32(1);int32(1);int32(1);int32(1);int32(1);int32(1);int32(1);int32(1);int32(1);int32(1);int32(1);int32(1);int32(1);int32(1);int32(1);int32(1);int32(1);int32(1);int32(1);int32(1);int32(1);int32(1);int32(1);int32(1);int32(1);int32(1);int32(1)]')  MultiplexValues=str2num('[double(0);double(0);double(0);double(0);double(0);double(0);double(0);double(0);double(0);double(0);double(0);double(0);double(0);double(0);double(0);double(0);double(0);double(0);double(0);double(0);double(0);double(0);double(0);double(0);double(0);double(0);double(0);double(0);double(0);double(0);double(0);double(0)]')  Factors=str2num('[double(1);double(0.05);double(0.01);double(1);double(0.05);double(0.01);double(1);double(0.05);double(0.01);double(1);double(0.05);double(0.01);double(1);double(0.05);double(0.01);double(1);double(0.05);double(0.01);double(1);double(0.05);double(0.01);double(1);double(0.05);double(0.01);double(1);double(0.05);double(0.01);double(1);double(0.05);double(0.01);double(1);double(1)]')  Offsets=str2num('[double(0);double(-400);double(-80);double(0);double(-400);double(-80);double(0);double(-400);double(-80);double(0);double(-400);double(-80);double(0);double(-400);double(-80);double(0);double(-400);double(-80);double(0);double(-400);double(-80);double(0);double(-400);double(-80);double(0);double(-400);double(-80);double(0);double(-400);double(-80);double(0);double(0)]')  Minimums=str2num('[double(0);double(-Inf);double(-Inf);double(0);double(-Inf);double(-Inf);double(0);double(-Inf);double(-Inf);double(0);double(-Inf);double(-Inf);double(0);double(-Inf);double(-Inf);double(0);double(-Inf);double(-Inf);double(0);double(-Inf);double(-Inf);double(0);double(-Inf);double(-Inf);double(0);double(-Inf);double(-Inf);double(0);double(-Inf);double(-Inf);double(0);double(0)]')  Maximums=str2num('[double(Inf);double(Inf);double(Inf);double(Inf);double(Inf);double(Inf);double(Inf);double(Inf);double(Inf);double(Inf);double(Inf);double(Inf);double(Inf);double(Inf);double(Inf);double(Inf);double(Inf);double(Inf);double(Inf);double(Inf);double(Inf);double(Inf);double(Inf);double(Inf);double(Inf);double(Inf);double(Inf);double(Inf);double(Inf);double(Inf);double(Inf);double(Inf)]')  Remote=off  ApplyMinMax=off  BRSSwitch=off
      settings: SourceProductName=Simulink Real-Time  DataFormat=manually specified signals
  S-Function1 : S-Function  FunctionName=NSTC297CANFDTransmitBlkLib  Parameters=|  SFunctionDeploymentMode=off  EnableBusSupport=off  mask(NSTC297 CANFD Transmit){Ns_DeviceID=ADAS Control Unit Gen2, Ns_ChannelNum=3, Ns_FrameType=CANFD, Ns_FrameBufferSize=0, Ns_OverflowCntOutFlg=off, Ns_SampleTime=-1}
      | uint16(Ns_DeviceID),
      | uint16(Ns_ChannelNum),
      | uint16(Ns_FrameType),
      | uint16(Ns_FrameBufferSize),
      | uint8(Ns_OverflowCntOutFlg),
      | double(Ns_SampleTime)
      mask prompts: Ns_DeviceID "Device:"; Ns_ChannelNum "Channel number:"; Ns_FrameType "Frame type:"; Ns_FrameBufferSize "Frame buffer size:"; Ns_OverflowCntOutFlg "Overflow count output"; Ns_SampleTime "Sample time:"
      mask init:
      | NSTC297CANFDTransmit_callback('portlabels');
      mask TypeOptions Ns_DeviceID: General Control Unit Gen2 | ADAS Control Unit Gen2
      mask TypeOptions Ns_ChannelNum: 0 | 1 | 2 | 3 | 4 | 5
      mask TypeOptions Ns_FrameType: CAN | CANFD
      mask Display: color('blue');text(0.98,0.9,'NovSteeds TC297','horizontalAlignment','right');color('blue');text(0.5,0.65,'CANFD Transmit','horizontalAlignment','center');color('black');text(0.5,0.35,'Type: CANFD','horizontalAlignment','center');text(0.5,0.50,'Channel: 3','horizontalAlignment','center');port_label('input',1, 'Msg');
  wires:
  Bus Selector13/1 -> CAN FD Pack1/1  "<Id_S0_001>"
  Bus Selector17/3 -> CAN FD Pack1/9  "<YPos_S0_003>"
  Bus Selector21/3 -> CAN FD Pack1/30  "<YPos_S0_010>"
  Bus Selector14/3 -> CAN FD Pack1/24  "<YPos_S0_008>"
  Bus Selector23/1 -> CAN FD Pack1/19  "<Id_S0_007>"
  Bus Selector14/2 -> CAN FD Pack1/23  "<XPos_S0_008>"
  Bus Selector15/2 -> CAN FD Pack1/26  "<XPos_S0_009>"
  Bus Selector16/2 -> CAN FD Pack1/5  "<XPos_S0_002>"
  Bus Selector22/1 -> CAN FD Pack1/16  "<Id_S0_006>"
  Bus Selector19/1 -> CAN FD Pack1/13  "<Id_S0_005>"
  Bus Selector13/3 -> CAN FD Pack1/3  "<YPos_S0_001>"
  Bus Selector21/2 -> CAN FD Pack1/29  "<XPos_S0_010>"
  Bus Selector22/3 -> CAN FD Pack1/18  "<YPos_S0_006>"
  Bus Selector23/3 -> CAN FD Pack1/21  "<YPos_S0_007>"
  Bus Selector15/1 -> CAN FD Pack1/25  "<Id_S0_009>"
  Bus Selector19/2 -> CAN FD Pack1/14  "<XPos_S0_005>"
  Bus Selector21/1 -> CAN FD Pack1/28  "<Id_S0_010>"
  Bus Selector15/3 -> CAN FD Pack1/27  "<YPos_S0_009>"
  Bus Selector12/10 -> Bus Selector21/1  "<M41ObjInfo>"
  Bus Selector20/1 -> CAN FD Pack1/31  "<NumberOfObjects_S3>"
  Bus Selector22/2 -> CAN FD Pack1/17  "<XPos_S0_006>"
  Bus Selector19/3 -> CAN FD Pack1/15  "<YPos_S0_005>"
  Bus Selector12/8 -> Bus Selector14/1  "<M31ObjInfo>"
  Bus Selector18/3 -> CAN FD Pack1/12  "<YPos_S0_004>"
  Bus Selector12/2 -> Bus Selector16/1  "<M01ObjInfo>"
  Bus Selector12/1 -> Bus Selector13/1  "<M00ObjInfo>"
  Bus Selector17/1 -> CAN FD Pack1/7  "<Id_S0_003>"
  Bus Selector12/3 -> Bus Selector17/1  "<M10ObjInfo>"
  Bus Selector17/2 -> CAN FD Pack1/8  "<XPos_S0_003>"
  Bus Selector23/2 -> CAN FD Pack1/20  "<XPos_S0_007>"
  Bus Selector12/4 -> Bus Selector18/1  "<M11ObjInfo>"
  Bus Selector18/2 -> CAN FD Pack1/11  "<XPos_S0_004>"
  Bus Selector12/11 -> Bus Selector20/1  "<FRRdr_bsCmnInfo>"
  Bus Selector14/1 -> CAN FD Pack1/22  "<Id_S0_008>"
  Bus Selector16/3 -> CAN FD Pack1/6  "<YPos_S0_002>"
  Bus Selector18/1 -> CAN FD Pack1/10  "<Id_S0_004>"
  Bus Selector16/1 -> CAN FD Pack1/4  "<Id_S0_002>"
  In1/1 -> Bus Selector12/1
  Bus Selector12/9 -> Bus Selector15/1  "<M40ObjInfo>"
  CAN FD Pack1/1 -> S-Function1/1
  Bus Selector12/6 -> Bus Selector22/1  "<M21ObjInfo>"
  Bus Selector12/5 -> Bus Selector19/1  "<M20ObjInfo>"
  Bus Selector12/7 -> Bus Selector23/1  "<M30ObjInfo>"
  Bus Selector13/2 -> CAN FD Pack1/2  "<XPos_S0_001>"

== system DFADAS2_SenFus_v1_201204RC_training_210115/Signal Input (Input)/Signal Input (50ms) (Input50)/RdrFrt/CmrInfo ==
  Bus Creator1 : BusCreator  Inputs=3
  Constant4 : Constant  Value=0.3
  Constant5 : Constant  Value=0.3
  Constant6 : Constant  Value=0.3
  Out1 : Outport
  wires:
  Bus Creator1/1 -> Out1/1  "VehInfo"
  Constant6/1 -> Bus Creator1/3
  Constant5/1 -> Bus Creator1/2
  Constant4/1 -> Bus Creator1/1

== system DFADAS2_SenFus_v1_201204RC_training_210115/Signal Input (Input)/Signal Input (50ms) (Input50)/RdrFrt/Rdr1 ==
  Bus Creator1 : BusCreator  Inputs=3
  Constant4 : Constant  Value=0.3
  Constant5 : Constant  Value=0.3
  Constant6 : Constant  Value=0.3
  Out1 : Outport
  wires:
  Bus Creator1/1 -> Out1/1  "VehInfo"
  Constant6/1 -> Bus Creator1/3
  Constant5/1 -> Bus Creator1/2
  Constant4/1 -> Bus Creator1/1

== system DFADAS2_SenFus_v1_201204RC_training_210115/Signal Input (Input)/Signal Input (50ms) (Input50)/Rear Left Radar(S0) Objects Information (RLRdr)/S0 Data Frame Read ==
  note: 目标：
      | ① 将可见的数据帧全部读出；
      | ② 仅对最新可见VF的数据帧进行数据解析。
      |
      | 首先将旧VF帧读完（不解析），然后进行RemainderCnt+1次的读取。最后一次读取的数据不解析，用于为未收到信号的通道置零。
  HFVFCnt : Inport
  IC : Inport  Port=2
  ObjectNum : Inport  Port=3
  Compare To Constant : simulink/Logic and Bit Operations/Compare To Constant  relop=>  const=0  OutDataTypeStr=boolean
  Enabled Subsystem : Subsystem  TreatAsAtomicUnit=on
  Logical Operator1 : Logic  Operator=OR  AllPortsSameDT=off  OutDataTypeStr=boolean
  Logical Operator3 : Logic  AllPortsSameDT=off  OutDataTypeStr=boolean
  Relational Operator3 : RelationalOperator  Operator===  OutDataTypeStr=boolean  RndMeth=Simplest
  S-Function200 : S-Function  FunctionName=NSTC297CANFDReceiveBlkLib  Parameters=|  SFunctionDeploymentMode=off  EnableBusSupport=off  mask(NSTC297 CANFD Receive){Ns_DeviceID=General Control Unit Gen2, Ns_ChannelNum=2, Ns_FrameID=849, Ns_IsVirtualFrame=on, Ns_RoleInVirtualFrame=Data Frame, Ns_HeaderFrameID=848, Ns_VirtualFrameStatusFlg=off, Ns_IncompleteFrameCntFlg=off, Ns_OverflowCntFlg=off, Ns_FrameBufferSize=5, Ns_SampleTime=-1}
      | uint16(Ns_DeviceID),
      | uint16(Ns_ChannelNum),
      | uint32(Ns_FrameID),
      | uint8(Ns_IsVirtualFrame),
      | uint16(Ns_RoleInVirtualFrame),
      | uint32(Ns_HeaderFrameID),
      | uint8(Ns_VirtualFrameStatusFlg),
      | uint8(Ns_IncompleteFrameCntFlg),
      | uint8(Ns_OverflowCntFlg),
      | uint16(Ns_FrameBufferSize),
      | double(Ns_SampleTime)
      mask prompts: Ns_DeviceID "Device:"; Ns_ChannelNum "Channel number:"; Ns_FrameID "Frame ID:"; Ns_IsVirtualFrame "Belong to a virtual frame"; Ns_RoleInVirtualFrame "Position in virtual frame:"; Ns_HeaderFrameID "Header frame ID:"; Ns_VirtualFrameStatusFlg "Current virtural frame status output"; Ns_IncompleteFrameCntFlg "Incomplete virtual frame count output"; Ns_OverflowCntFlg "Overflow count output"; Ns_FrameBufferSize "Frame buffer size:"; Ns_SampleTime "Sample time:"
      mask init:
      | NSTC297CANFDReceive_callback('portlabels');
      mask TypeOptions Ns_DeviceID: General Control Unit Gen2 | ADAS Control Unit Gen2
      mask TypeOptions Ns_ChannelNum: 0 | 1 | 2 | 3 | 4 | 5
      mask Callback Ns_IsVirtualFrame: NSTC297CANFDReceive_callback('Belong to a virtual frame');
      mask TypeOptions Ns_RoleInVirtualFrame: Header Frame | Data Frame | Trailer Frame
      mask Callback Ns_RoleInVirtualFrame: NSTC297CANFDReceive_callback('Position in virtual frame');
      mask Display: color('blue');text(0.02,0.9,'NovSteeds TC297','horizontalAlignment','left');color('blue');text(0.5,0.7,'CANFD Receive','horizontalAlignment','center');color('black');text(0.5,0.6,'Channel: 2','horizontalAlignment','center');text(0.5,0.5,'ID: 849','horizontalAlignment','center');text(0.5,0.4,'Virtual Frame: Data Frame','horizontalAlignment','center');port_label('output',1, 'VFCnt');port_label('output',2, 'RemainderCnt');port_label('output',3, 'Msg');
  Subsystem : Subsystem
  Switch : Switch  Criteria=u2 > Threshold
  VsblMnmt : Subsystem
  While Iterator : WhileIterator  MaxIters=10  ResetStates=reset
  RLRdr_bsObjInfo : Outport
  wires:
  IC/1 -> While Iterator/2
  S-Function200/3 -> Enabled Subsystem/2(Msg)
  S-Function200/2 -> Compare To Constant/1, Enabled Subsystem/1(RemainderCnt)
  S-Function200/1 -> VsblMnmt/2(LocVFCnt), Relational Operator3/2
  HFVFCnt/1 -> VsblMnmt/1(HFVFCnt), Relational Operator3/1
  VsblMnmt/1(EnFlg) -> Logical Operator1/1
  Logical Operator1/1 -> While Iterator/1
  Relational Operator3/1 -> Logical Operator3/1
  Compare To Constant/1 -> Logical Operator3/2
  Enabled Subsystem/1(RLRdrObjInfo) -> Switch/1
  Subsystem/1(RLRdrObjInfo) -> Switch/3
  Logical Operator3/1 -> Logical Operator1/2, Enabled Subsystem/Enable
  ObjectNum/1 -> Enabled Subsystem/3(obj_num), Switch/2
  Switch/1 -> RLRdr_bsObjInfo/1
